simulink model "sl_subsys_fcncallerr9"  (Simulink 6.0)
settings: Solver=FixedStepDiscrete  StartTime=0.0  StopTime=10.0  FixedStep=1  RelTol=1e-3
settings Model: CovMetricSettings=d  Creator=The MathWorks Inc.  LastModifiedBy=batserve  ExtModeAutoUpdateStatusClock=off
settings OptimizationCC: BlockReduction=off  BooleanDataType=off
settings DebuggingCC: CheckExecutionContextPreStartOutputMsg=on  CheckExecutionContextRuntimeOutputMsg=on  SolverPrmCheckMsg=none  UnconnectedInputMsg=none  UnconnectedOutputMsg=none  UnconnectedLineMsg=none
settings HardwareCC: TargetUnknown=on

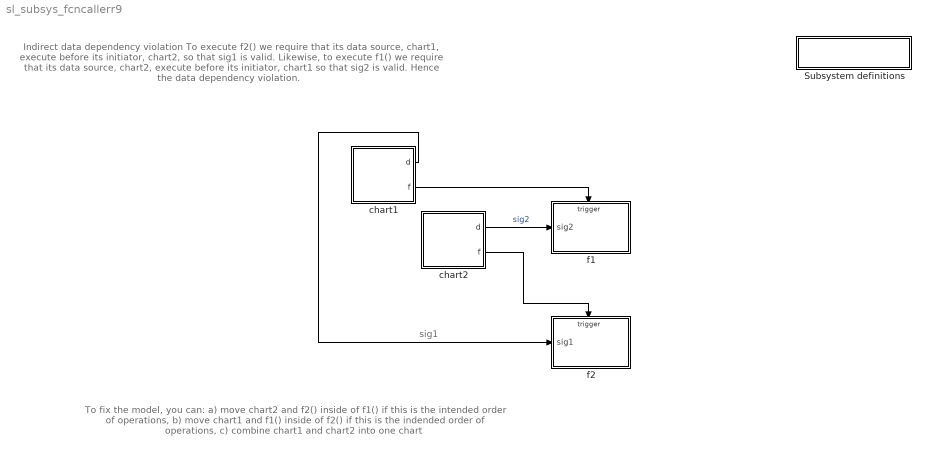
== system sl_subsys_fcncallerr9 ==
  note: Indirect data dependency violation
      |
      | To execute f2() we require that its data source, chart1,
      | execute before its initiator, chart2, so that sig1 is
      | valid. Likewise, to execute f1() we require that its data
      | source, chart2, execute before its initiator, chart1 so that
      | sig2 is valid. Hence the data dependency violation.
  note: To fix the model, you can:
      | a) move chart2 and f2() inside of f1() if this is the intended order of operations,
      | b) move chart1 and f1() inside of f2() if this is the indended order of operations,
      | c) combine chart1 and chart2 into one chart
  note: sig1
  " Subsystem definitions" : Subsystem  PropExecContextAcrossSSBoundary=on
      settings: OpenFcn=helpview([matlabroot,'/toolbox/simulink/simdemos/sl_subsys_definitions.html']);
      mask Display: disp('Subsystem\ndefinitions')
  chart1 : Stateflow chart  PropExecContextAcrossSSBoundary=on
  chart2 : Stateflow chart  PropExecContextAcrossSSBoundary=on
  f1 : Subsystem  TreatAsAtomicUnit=on  PropExecContextAcrossSSBoundary=on
  f2 : Subsystem  TreatAsAtomicUnit=on  PropExecContextAcrossSSBoundary=on
  wires:
  chart1/2(f) -> f1/Trigger
  chart1/1(d) -> f2/1(sig1)
  chart2/1(d) -> f1/1(sig2)  "sig2"
  chart2/2(f) -> f2/Trigger

== system sl_subsys_fcncallerr9/ Subsystem definitions ==

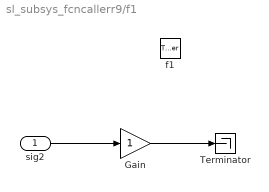
== system sl_subsys_fcncallerr9/f1 ==
  sig2 : Inport  Port=1  LatchInput=off
  f1 : TriggerPort  TriggerType=function-call
  Gain : Gain  SaturateOnIntegerOverflow=on
  Terminator : Terminator
  wires:
  sig2/1 -> Gain/1
  Gain/1 -> Terminator/1

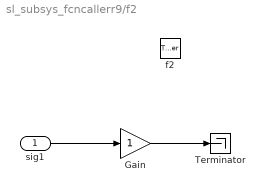
== system sl_subsys_fcncallerr9/f2 ==
  sig1 : Inport  Port=1  LatchInput=off
  f2 : TriggerPort  TriggerType=function-call
  Gain : Gain  SaturateOnIntegerOverflow=on
  Terminator : Terminator
  wires:
  sig1/1 -> Gain/1
  Gain/1 -> Terminator/1

== stateflow chart chart2 ==
  state one/
    entry: f; d=1;
  state two/
    entry: f; d=2;
  one -> two
  two -> one
  (default) -> one
  data: d output double
  events: f output FUNCTION_CALL_EVENT

== stateflow chart chart1 ==
  state one/
    entry: f; d=1;
  state two/
    entry: f; d=2;
  one -> two
  two -> one
  (default) -> one
  data: d output double
  events: f output FUNCTION_CALL_EVENT
